simulink model "sampleModel53"  (R2021b)
settings: Solver=VariableStepAuto  StartTime=0.0  StopTime=10.0  RelTol=1e-3
undefined symbols (not defined in the file or in its folder): DiscIntNeverNeededParam, magnitude, Newton, Raphson
libraries: simulink x11, slpidlib x1
settings Model: Creator=user  LastModifiedBy=user

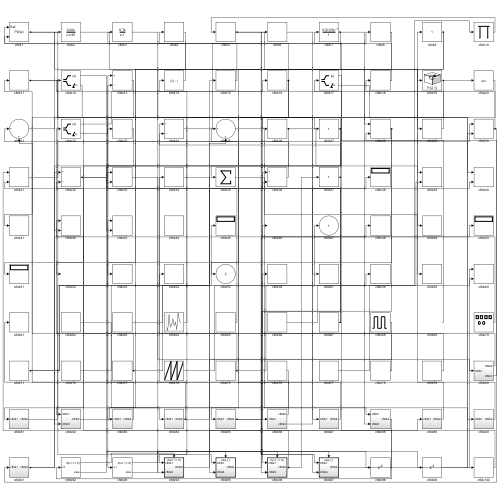
[thumbnail: Simulink's stored preview of the top-level diagram]
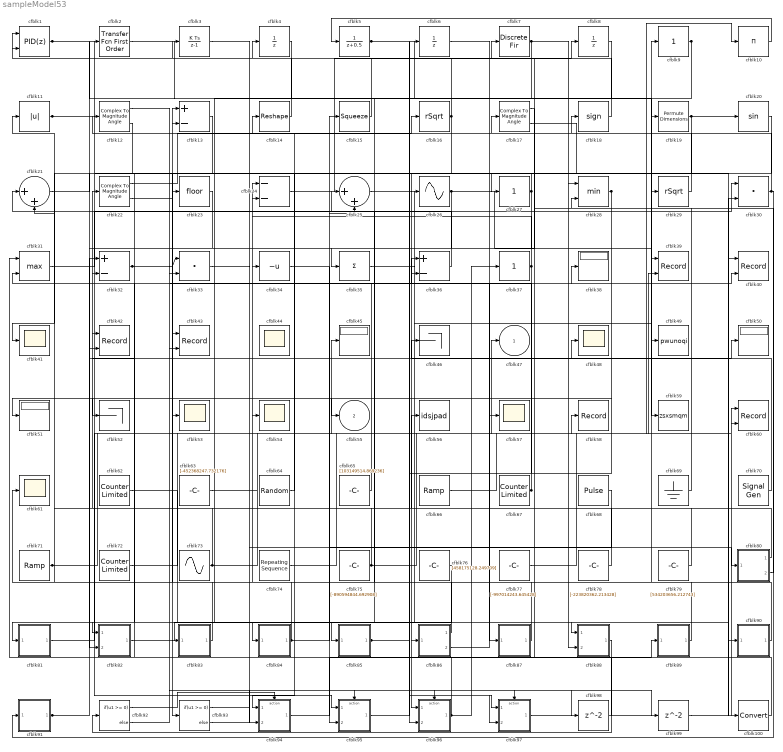
== system sampleModel53 ==
  cfblk1 : slpidlib/PID Controller (2DOF)  Controller=PID  Form=Parallel  TimeDomain=Discrete-time  UseExternalTs=off  SampleTime=1  IntegratorMethod=Forward Euler  FilterMethod=Forward Euler  ControllerParametersSource=internal  P=1  I=1  D=0  UseFilter=on  N=100  b=1  c=1  TunerSelectOption=Transfer Function Based (PID Tuner App)  InitialConditionSource=internal  InitialConditionForIntegrator=0  InitialConditionForFilter=0  DifferentiatorICPrevScaledInput=0  ExternalReset=none  TrackingMode=off  Kt=1  LimitOutput=off  SatLimitsSource=internal  UpperSaturationLimit=inf  LowerSaturationLimit=-inf  LinearizeAsGain=off  AntiWindupMode=none  Kb=1  POutMin=[]  POutMax=[]  IOutMin=[]  IOutMax=[]  DOutMin=[]  DOutMax=[]  NOutMin=[]  NOutMax=[]  bOutMin=[]  bOutMax=[]  cOutMin=[]  cOutMax=[]  SumOutMin=[]  SumOutMax=[]  SaturationOutMin=[]  SaturationOutMax=[]  PParamMin=[]  PParamMax=[]  IParamMin=[]  IParamMax=[]  DParamMin=[]  DParamMax=[]  NParamMin=[]  NParamMax=[]  bParamMin=[]  bParamMax=[]  cParamMin=[]  cParamMax=[]  KbParamMin=[]  KbParamMax=[]  KtParamMin=[]  KtParamMax=[]  KbOutMin=[]  KbOutMax=[]  KtOutMin=[]  KtOutMax=[]  IntegratorOutMin=[]  IntegratorOutMax=[]  FilterOutMin=[]  FilterOutMax=[]  SumI1OutMin=[]  SumI1OutMax=[]  SumI2OutMin=[]  SumI2OutMax=[]  SumI3OutMin=[]  SumI3OutMax=[]  SumI4OutMin=[]  SumI4OutMax=[]  SumDOutMin=[]  SumDOutMax=[]  Sum1OutMin=[]  Sum1OutMax=[]  Sum2OutMin=[]  Sum2OutMax=[]  Sum3OutMin=[]  Sum3OutMax=[]  DifferentiatorOutMin=[]  DifferentiatorOutMax=[]  FilterDiffOutCoefMin=[]  FilterDiffOutCoefMax=[]  ReciprocalOutMin=[]  ReciprocalOutMax=[]  SumDenOutMin=[]  SumDenOutMax=[]  SumNumOutMin=[]  SumNumOutMax=[]  DivideOutMin=[]  DivideOutMax=[]  UdiffTsProdOutMin=[]  UdiffTsProdOutMax=[]  NTsProdOutMin=[]  NTsProdOutMax=[]  UintegralTsProdOutMin=[]  UintegralTsProdOutMax=[]  UngainTsProdOutMin=[]  UngainTsProdOutMax=[]  IntegratorContinuousStateAttributes=''  IntegratorStateMustResolveToSignalObject=off  IntegratorRTWStateStorageClass=Auto  FilterContinuousStateAttributes=''  FilterStateMustResolveToSignalObject=off  FilterRTWStateStorageClass=Auto  ParallelPVariant=InternalParameters  IdealPVariant=Disabled  IVariant=InternalParameters  DVariant=InternalParameters  bVariant=InternalParameters  cVariant=InternalParameters  IntegratorVariant=Discrete  SatVariant=Disabled  AWVariant=Passthrough  PCopyVariant=Disabled  TRVariant=Disabled  FdbkBlocksVariant=Forward  IdealPFdbkVariant=Disabled  SatFdbkVariant=Disabled  DerivativeFilterVariant=ForwardEulerFilter  NVariant=InternalParameters  NCopyVariant=Disabled  FilterICVariant=InternalICsFilter  IntegratorICVariant=InternalICs  ExternalResetVariant=Disabled  TRSumVariant=Passthrough  SumFdbkVariant=Disabled  SumVariant=Sum_PID  TsampFilterVariant=InternalTs  TsampNgainVariant=Passthrough  TsampIntegralVariant=Passthrough  ExternalSaturationOutDataTypeStr=Inherit: Same as second input
      settings: SourceProductBaseCode=SL
  cfblk10 : Product  Inputs=*
  cfblk100 : DataTypeConversion
  cfblk11 : Abs
  cfblk12 : ComplexToMagnitudeAngle
  cfblk13 : Sum  Inputs=+-
  cfblk14 : Reshape
  cfblk15 : Squeeze
  cfblk16 : Sqrt  Operator=rSqrt  AlgorithmType=Newton-Raphson  SaturateOnIntegerOverflow=on
  cfblk17 : ComplexToMagnitudeAngle
  cfblk18 : Signum
  cfblk19 : PermuteDimensions
  cfblk2 : simulink/Discrete/Transfer Fcn First Order  PoleZ=0.95  ICPrevOutput=0.0  DoSatur=off
  cfblk20 : Trigonometry
  cfblk21 : Sum  Inputs=|++
  cfblk22 : ComplexToMagnitudeAngle
  cfblk23 : Rounding
  cfblk24 : Sum  Inputs=--
  cfblk25 : Sum  Inputs=|++
  cfblk26 : Sin  TimeSource=Use external signal  SampleTime=0
  cfblk27 : simulink/Math Operations/Slider Gain  gain=1  low=0  high=2
  cfblk28 : MinMax  Inputs=2
  cfblk29 : Sqrt  Operator=rSqrt  AlgorithmType=Newton-Raphson  SaturateOnIntegerOverflow=on
  cfblk3 : DiscreteIntegrator  ICPrevOutput=DiscIntNeverNeededParam  ICPrevScaledInput=DiscIntNeverNeededParam
  cfblk30 : DotProduct  InputSameDT=on  OutDataTypeStr=Inherit: Inherit via internal rule
  cfblk31 : MinMax  Function=max  Inputs=2
  cfblk32 : Sum  Inputs=+-
  cfblk33 : DotProduct  InputSameDT=on  OutDataTypeStr=Inherit: Inherit via internal rule
  cfblk34 : UnaryMinus
  cfblk35 : Sum  Inputs=+
  cfblk36 : Sum  Inputs=+-
  cfblk37 : simulink/Math Operations/Slider Gain  gain=1  low=0  high=2
  cfblk{38,45,50..51} (4 alike) : Display
  cfblk39 : Record  FileSettingsInternal="{\"entries\":[{\"content\":{\"excelSettings\":{\"content\":{},\"type\":\"Streamout.ExcelSettings\"}},\"type\":\"Streamout.FileSettingStorage\",\"uuid\":\"36555a3f-5799-4d89-b4f4-813525baae06\"}],\"packageUris\":[\"http://schema.mathworks.com/mf0/streamout_blocks/R2020a\"],\"version\":\"1.0\"}"  Layout=[1 1]  SignalsInternal="{\"entries\":[{\"content\":{\"signals\":[{\"content\":{\"blockPath\":[\"sampleModel53/cfblk39\"],\"channel\":[],\"dimensions\":[1],\"domain\":\"sampleModel53/cfblk39\",\"lineColor\":\"#a2142f\",\"plots\":[1],\"port\":1,\"sid\":[\"\"],\"signalID\":2017,\"signalName\":\"cfblk26\"},\"type\":\"RecordBlkView.Signal\",\"uuid\":\"47f0a369-7cc4-4aaa-9385-732514935d38\"},{\"content\":{\"blockPath\":[\"sampleModel53/cfblk39\"],\"channel\":[],\"dimensions\":[1],\"domain\":\"sampleModel53/cfblk39\",\"lineColor\":\"#139fff\",\"plots\":[1],\"port\":2,\"sid\":[\"\"],\"signalID\":2021,\"signalName\":\"cfblk75\"},\"type\":\"RecordBlkView.Signal\",\"uuid\":\"4d1bc853-d276-4e83-93c2-32a1ede8454b\"}]},\"type\":\"RecordBlkView.InputSignals\",\"uuid\":\"ef9d1d75-79a9-4377-b019-a30109193e72\"}],\"packageUris\":[\"http://schema.mathworks.com/mf0/streamout_blocks/R2020a\"],\"version\":\"1.0\"}"  VisualizationBindings="{\"xyplotplugin\":{\"info\":[{\"series\":[{\"bindingParametersList\":[{\"parameter\":\"X-Axis\",\"signalID\":2017,\"signalName\":\"cfblk26\"},{\"parameter\":\"Y-Axis\",\"signalID\":2021,\"signalName\":\"cfblk75\"}],\"seriesID\":35911}],\"subplotID\":1}]}}"  CompatibilityTag=XY
  cfblk4 : UnitDelay  HasFrameUpgradeWarning=on
  cfblk40 : Record  FileSettingsInternal="{\"entries\":[{\"content\":{\"excelSettings\":{\"content\":{},\"type\":\"Streamout.ExcelSettings\"}},\"type\":\"Streamout.FileSettingStorage\",\"uuid\":\"29f311e9-4cb5-4aae-ab6d-f238a6542dbf\"}],\"packageUris\":[\"http://schema.mathworks.com/mf0/streamout_blocks/R2020a\"],\"version\":\"1.0\"}"  Layout=[1 1]  SignalsInternal="{\"entries\":[{\"content\":{\"signals\":[{\"content\":{\"blockPath\":[\"sampleModel53/cfblk40\"],\"channel\":[],\"dimensions\":[1],\"domain\":\"sampleModel53/cfblk40\",\"lineColor\":\"#a2142f\",\"plots\":[1],\"port\":1,\"sid\":[\"\"],\"signalID\":2025,\"signalName\":\"cfblk11\"},\"type\":\"RecordBlkView.Signal\",\"uuid\":\"6599d64e-fdeb-4881-badc-896bf7f9b191\"},{\"content\":{\"blockPath\":[\"sampleModel53/cfblk40\"],\"channel\":[],\"dimensions\":[1],\"domain\":\"sampleModel53/cfblk40\",\"lineColor\":\"#139fff\",\"plots\":[1],\"port\":2,\"sid\":[\"\"],\"signalID\":2029,\"signalName\":\"cfblk32\"},\"type\":\"RecordBlkView.Signal\",\"uuid\":\"6d17c54a-5a2b-4875-95ea-40abd550d686\"}]},\"type\":\"RecordBlkView.InputSignals\",\"uuid\":\"16042054-2248-4dd5-be65-24b2471db457\"}],\"packageUris\":[\"http://schema.mathworks.com/mf0/streamout_blocks/R2020a\"],\"version\":\"1.0\"}"  VisualizationBindings="{\"xyplotplugin\":{\"info\":[{\"series\":[{\"bindingParametersList\":[{\"parameter\":\"X-Axis\",\"signalID\":2025,\"signalName\":\"cfblk11\"},{\"parameter\":\"Y-Axis\",\"signalID\":2029,\"signalName\":\"cfblk32\"}],\"seriesID\":247}],\"subplotID\":1}]}}"  CompatibilityTag=XY
  cfblk{41,44,48,53..54,57,61} (7 alike) : Scope
      cfblk44 settings: Floating=on
  cfblk42 : Record  FileSettingsInternal="{\"entries\":[{\"content\":{\"excelSettings\":{\"content\":{},\"type\":\"Streamout.ExcelSettings\"}},\"type\":\"Streamout.FileSettingStorage\",\"uuid\":\"2795f945-7d6f-4af1-afb2-df17c85014fd\"}],\"packageUris\":[\"http://schema.mathworks.com/mf0/streamout_blocks/R2020a\"],\"version\":\"1.0\"}"  Layout=[1 1]  SignalsInternal="{\"entries\":[{\"content\":{\"signals\":[{\"content\":{\"blockPath\":[\"sampleModel53/cfblk42\"],\"channel\":[],\"dimensions\":[1],\"domain\":\"sampleModel53/cfblk42\",\"lineColor\":\"#a2142f\",\"plots\":[1],\"port\":1,\"sid\":[\"\"],\"signalID\":2033,\"signalName\":\"cfblk96\"},\"type\":\"RecordBlkView.Signal\",\"uuid\":\"f70ba7eb-dc46-4726-8912-a281d005d84a\"},{\"content\":{\"blockPath\":[\"sampleModel53/cfblk42\"],\"channel\":[],\"dimensions\":[1],\"domain\":\"sampleModel53/cfblk42\",\"lineColor\":\"#139fff\",\"plots\":[1],\"port\":2,\"sid\":[\"\"],\"signalID\":2037,\"signalName\":\"cfblk27\"},\"type\":\"RecordBlkView.Signal\",\"uuid\":\"e8cdc3a5-91fa-4319-be48-d51676adf6e4\"}]},\"type\":\"RecordBlkView.InputSignals\",\"uuid\":\"f027bfeb-bbc1-4bf5-989f-a466d2fc895d\"}],\"packageUris\":[\"http://schema.mathworks.com/mf0/streamout_blocks/R2020a\"],\"version\":\"1.0\"}"  VisualizationBindings="{\"xyplotplugin\":{\"info\":[{\"series\":[{\"bindingParametersList\":[{\"parameter\":\"X-Axis\",\"signalID\":2033,\"signalName\":\"cfblk96\"},{\"parameter\":\"Y-Axis\",\"signalID\":2037,\"signalName\":\"cfblk27\"}],\"seriesID\":22493}],\"subplotID\":1}]}}"  CompatibilityTag=XY
  cfblk43 : Record  FileSettingsInternal="{\"entries\":[{\"content\":{\"excelSettings\":{\"content\":{},\"type\":\"Streamout.ExcelSettings\"}},\"type\":\"Streamout.FileSettingStorage\",\"uuid\":\"262fdbcb-1a99-4405-9c28-3705634d857c\"}],\"packageUris\":[\"http://schema.mathworks.com/mf0/streamout_blocks/R2020a\"],\"version\":\"1.0\"}"  Layout=[1 1]  SignalsInternal="{\"entries\":[{\"content\":{\"signals\":[{\"content\":{\"blockPath\":[\"sampleModel53/cfblk43\"],\"channel\":[],\"dimensions\":[1],\"domain\":\"sampleModel53/cfblk43\",\"lineColor\":\"#a2142f\",\"plots\":[1],\"port\":1,\"sid\":[\"\"],\"signalID\":2041,\"signalName\":\"cfblk71\"},\"type\":\"RecordBlkView.Signal\",\"uuid\":\"31af7c79-9017-45d5-9c95-6f76501c4ed0\"},{\"content\":{\"blockPath\":[\"sampleModel53/cfblk43\"],\"channel\":[],\"dimensions\":[1],\"domain\":\"sampleModel53/cfblk43\",\"lineColor\":\"#139fff\",\"plots\":[1],\"port\":2,\"sid\":[\"\"],\"signalID\":2045,\"signalName\":\"cfblk26\"},\"type\":\"RecordBlkView.Signal\",\"uuid\":\"6227f1e4-0aa9-438c-91b2-f1da6c01766f\"}]},\"type\":\"RecordBlkView.InputSignals\",\"uuid\":\"4e3f22c6-0fd5-443b-ac92-023e98c5f6af\"}],\"packageUris\":[\"http://schema.mathworks.com/mf0/streamout_blocks/R2020a\"],\"version\":\"1.0\"}"  VisualizationBindings="{\"xyplotplugin\":{\"info\":[{\"series\":[{\"bindingParametersList\":[{\"parameter\":\"X-Axis\",\"signalID\":2041,\"signalName\":\"cfblk71\"},{\"parameter\":\"Y-Axis\",\"signalID\":2045,\"signalName\":\"cfblk26\"}],\"seriesID\":22878}],\"subplotID\":1}]}}"  CompatibilityTag=XY
  cfblk46 : Terminator
  cfblk49 : ToWorkspace  VariableName=pwunoqi  SaveFormat=Timeseries  SampleTime=-1
  cfblk5 : DiscreteTransferFcn  SampleTime=1
  cfblk52 : Terminator
  cfblk56 : ToWorkspace  VariableName=idsjpad  SaveFormat=Timeseries  SampleTime=-1
  cfblk58 : Record  FileSettingsInternal="{\"entries\":[{\"content\":{\"excelSettings\":{\"content\":{},\"type\":\"Streamout.ExcelSettings\"}},\"type\":\"Streamout.FileSettingStorage\",\"uuid\":\"e85a456c-a740-4745-ba77-d61e779d1d41\"}],\"packageUris\":[\"http://schema.mathworks.com/mf0/streamout_blocks/R2020a\"],\"version\":\"1.0\"}"  SignalsInternal="{\"entries\":[{\"content\":{\"signals\":[{\"content\":{\"blockPath\":[\"sampleModel53/cfblk58\"],\"channel\":[],\"dimensions\":[1,1],\"domain\":\"sampleModel53/cfblk58\",\"lineColor\":\"#0072bd\",\"plots\":[1],\"port\":1,\"sid\":[\"\"],\"signalID\":2049,\"signalName\":\"cfblk85\"},\"type\":\"RecordBlkView.Signal\",\"uuid\":\"17db5c15-ca79-42f1-988a-ac83bc16403a\"}]},\"type\":\"RecordBlkView.InputSignals\",\"uuid\":\"5543be3e-2cf2-4ad7-9ef1-191d5603f8b7\"}],\"packageUris\":[\"http://schema.mathworks.com/mf0/streamout_blocks/R2020a\"],\"version\":\"1.0\"}"  VisualizationBindings="{\"sparklinesplugin\":{\"info\":[{\"bindingParametersList\":[],\"subplotID\":1}]}}"
  cfblk59 : ToWorkspace  VariableName=zsxsmqm  SaveFormat=Timeseries  SampleTime=-1
  cfblk6 : UnitDelay  HasFrameUpgradeWarning=on
  cfblk60 : Record  FileSettingsInternal="{\"entries\":[{\"content\":{\"excelSettings\":{\"content\":{},\"type\":\"Streamout.ExcelSettings\"}},\"type\":\"Streamout.FileSettingStorage\",\"uuid\":\"266a0de7-ebb2-40d2-bb8b-a752c9a132df\"}],\"packageUris\":[\"http://schema.mathworks.com/mf0/streamout_blocks/R2020a\"],\"version\":\"1.0\"}"  Layout=[1 1]  SignalsInternal="{\"entries\":[{\"content\":{\"signals\":[{\"content\":{\"blockPath\":[\"sampleModel53/cfblk60\"],\"channel\":[],\"dimensions\":[1,1],\"domain\":\"sampleModel53/cfblk60\",\"lineColor\":\"#a2142f\",\"plots\":[1],\"port\":1,\"sid\":[\"\"],\"signalID\":2053,\"signalName\":\"cfblk97\"},\"type\":\"RecordBlkView.Signal\",\"uuid\":\"49a729a9-27c5-4996-8fdc-6a282c899358\"},{\"content\":{\"blockPath\":[\"sampleModel53/cfblk60\"],\"channel\":[],\"dimensions\":[1],\"domain\":\"sampleModel53/cfblk60\",\"lineColor\":\"#139fff\",\"plots\":[1],\"port\":2,\"sid\":[\"\"],\"signalID\":2057,\"signalName\":\"cfblk66\"},\"type\":\"RecordBlkView.Signal\",\"uuid\":\"6ac5d0f1-1282-4ff0-ab72-565fc0b345a4\"}]},\"type\":\"RecordBlkView.InputSignals\",\"uuid\":\"cdacac38-5788-4d0c-a38f-7dc9b2a02f40\"}],\"packageUris\":[\"http://schema.mathworks.com/mf0/streamout_blocks/R2020a\"],\"version\":\"1.0\"}"  VisualizationBindings="{\"xyplotplugin\":{\"info\":[{\"series\":[{\"bindingParametersList\":[{\"parameter\":\"X-Axis\",\"signalID\":2053,\"signalName\":\"cfblk97\"},{\"parameter\":\"Y-Axis\",\"signalID\":2057,\"signalName\":\"cfblk66\"}],\"seriesID\":18023}],\"subplotID\":1}]}}"  CompatibilityTag=XY
  cfblk62 : simulink/Sources/Counter Limited  uplimit=[412.000000]  tsamp=-1
  cfblk63 : Constant  Value=[-452368247.732176]  SampleTime=1
  cfblk64 : UniformRandomNumber  Minimum=[-947621677.396505]  Maximum=[4577245631.312114]  Seed=[41948386.000000]  SampleTime=0.1
  cfblk65 : Constant  Value=[103149514.869236]  SampleTime=1
  cfblk66 : simulink/Sources/Ramp  slope=[-8825.450027]  start=[23.823209]  InitialOutput=[549085.262431]
  cfblk67 : simulink/Sources/Counter Limited  uplimit=[704.000000]  tsamp=-1
  cfblk68 : DiscretePulseGenerator  PulseType=Time based  Amplitude=[352690679.292892]  Period=[77561653.661700]  PulseWidth=5  PhaseDelay=[5.000000]
  cfblk69 : Ground
  cfblk7 : DiscreteFir  SampleTime=1
  cfblk70 : SignalGenerator  WaveForm=sawtooth  Amplitude=[-548495900.306508]
  cfblk71 : simulink/Sources/Ramp  slope=[4666.478299]  start=[41.983300]  InitialOutput=[189060.018572]
  cfblk72 : simulink/Sources/Counter Limited  uplimit=[395.000000]  tsamp=-1
  cfblk73 : Sin  Amplitude=[236450243.117325]  Bias=[354333946.592346]  SampleTime=0
  cfblk74 : simulink/Sources/Repeating Sequence  rep_seq_t=[0 2]  rep_seq_y=[-965358426.288802, 477876210.954182]
  cfblk75 : Constant  Value=[-890594844.692908]  SampleTime=1
  cfblk76 : Constant  Value=[458175128.249709]  SampleTime=1
  cfblk77 : Constant  Value=[-997014243.645428]  SampleTime=1
  cfblk78 : Constant  Value=[-223820362.213428]  SampleTime=1
  cfblk79 : Constant  Value=[534203656.212743]  SampleTime=1
  cfblk8 : UnitDelay  HasFrameUpgradeWarning=on
  cfblk80 : Subsystem
  cfblk81 : Subsystem
  cfblk82 : Subsystem
  cfblk83 : Subsystem
  cfblk84 : Subsystem
  cfblk85 : Subsystem
  cfblk86 : Subsystem
  cfblk87 : Subsystem
  cfblk88 : Subsystem
  cfblk89 : Subsystem
  cfblk9 : simulink/Math Operations/Slider Gain  gain=1  low=0  high=2
  cfblk90 : Subsystem
  cfblk91 : Subsystem
  cfblk92 : If  IfExpression=u1 >= 0  SampleTime=1
  cfblk93 : If  IfExpression=u1 >= 0  SampleTime=1
  cfblk94 : Subsystem  TreatAsAtomicUnit=on
  cfblk95 : Subsystem  TreatAsAtomicUnit=on
  cfblk96 : Subsystem  TreatAsAtomicUnit=on
  cfblk97 : Subsystem  TreatAsAtomicUnit=on
  cfblk98 : Delay  SampleTime=1
  cfblk99 : Delay  SampleTime=1
  cfblk47 : Outport
  cfblk55 : Outport  Port=2
  wires:
  cfblk11/1 -> cfblk95/1(cfblk1), cfblk40/1
  cfblk89/1(cfblk2) -> cfblk9/1
  cfblk77/1 -> cfblk10/1
  cfblk9/1 -> cfblk59/1, cfblk53/1
  cfblk16/1 -> cfblk96/1(cfblk1), cfblk52/1, cfblk1/2, cfblk94/1(cfblk1)
  cfblk36/1 -> cfblk21/1
  cfblk75/1 -> cfblk24/1, cfblk39/2
  cfblk74/1 -> cfblk47/1
  cfblk24/1 -> cfblk8/1
  cfblk88/1(cfblk2) -> cfblk92/1
  cfblk35/1 -> cfblk49/1
  cfblk82/1(cfblk2) -> cfblk84/1(cfblk1)
  cfblk67/1 -> cfblk13/1, cfblk36/1
  cfblk76/1 -> cfblk81/1(cfblk1)
  cfblk14/1 -> cfblk1/1
  cfblk31/1 -> cfblk30/1
  cfblk94/1(cfblk2) -> cfblk89/1(cfblk1)
  cfblk73/1 -> cfblk45/1, cfblk32/2
  cfblk25/1 -> cfblk88/1(cfblk1)
  cfblk13/1 -> cfblk93/1
  cfblk28/1 -> cfblk96/2(cfblk5), cfblk51/1
  cfblk79/1 -> cfblk22/1
  cfblk26/1 -> cfblk39/1, cfblk43/2
  cfblk4/1 -> cfblk83/1(cfblk1)
  cfblk7/1 -> cfblk28/1, cfblk94/2(cfblk4)
  cfblk2/1 -> cfblk88/2(cfblk3)
  cfblk29/1 -> cfblk18/1
  cfblk37/1 -> cfblk86/1(cfblk1), cfblk24/2
  cfblk22/1 -> cfblk16/1
  cfblk1/1 -> cfblk87/1(cfblk1), cfblk19/1
  cfblk83/1(cfblk2) -> cfblk13/2
  cfblk64/1 -> cfblk14/1
  cfblk90/1(cfblk2) -> cfblk25/1
  cfblk97/1(cfblk2) -> cfblk60/1
  cfblk27/1 -> cfblk55/1, cfblk42/2, cfblk26/1
  cfblk30/1 -> cfblk91/1(cfblk1), cfblk12/1
  cfblk15/1 -> cfblk3/1
  cfblk5/1 -> cfblk29/1, cfblk97/2(cfblk4)
  cfblk87/1(cfblk2) -> cfblk61/1
  cfblk18/1 -> cfblk4/1
  cfblk69/1 -> cfblk7/1
  cfblk8/1 -> cfblk35/1
  cfblk80/1(cfblk2) -> cfblk56/1
  cfblk71/1 -> cfblk15/1, cfblk43/1
  cfblk85/1(cfblk2) -> cfblk58/1, cfblk97/1(cfblk1)
  cfblk84/1(cfblk2) -> cfblk31/2, cfblk36/2
  cfblk10/1 -> cfblk5/1
  cfblk66/1 -> cfblk60/2
  cfblk19/1 -> cfblk85/1(cfblk1), cfblk20/1
  cfblk6/1 -> cfblk57/1
  cfblk12/2 -> cfblk41/1
  cfblk22/2 -> cfblk23/1
  cfblk72/1 -> cfblk25/2
  cfblk95/1(cfblk2) -> cfblk50/1
  cfblk70/1 -> cfblk46/1
  cfblk32/1 -> cfblk33/1, cfblk40/2
  cfblk86/1(cfblk2) -> cfblk34/1
  cfblk91/1(cfblk2) -> cfblk32/1, cfblk48/1
  cfblk81/1(cfblk2) -> cfblk54/1
  cfblk23/1 -> cfblk82/1(cfblk1)
  cfblk21/1 -> cfblk2/1
  cfblk78/1 -> cfblk11/1
  cfblk68/1 -> cfblk95/2(cfblk4)
  cfblk17/1 -> cfblk33/2
  cfblk80/2(cfblk3) -> cfblk28/2
  cfblk86/2(cfblk4) -> cfblk38/1
  cfblk3/1 -> cfblk27/1
  cfblk33/1 -> cfblk80/1(cfblk1)
  cfblk65/1 -> cfblk21/2
  cfblk96/1(cfblk2) -> cfblk42/1, cfblk37/1
  cfblk63/1 -> cfblk6/1
  cfblk17/2 -> cfblk90/1(cfblk1)
  cfblk20/1 -> cfblk82/2(cfblk5)
  cfblk92/1 -> cfblk94/Action
  cfblk92/2 -> cfblk95/Action
  cfblk93/1 -> cfblk96/Action
  cfblk93/2 -> cfblk97/Action
  cfblk34/1 -> cfblk98/1
  cfblk98/1 -> cfblk31/1
  cfblk12/1 -> cfblk99/1
  cfblk99/1 -> cfblk30/2
  cfblk62/1 -> cfblk100/1
  cfblk100/1 -> cfblk17/1

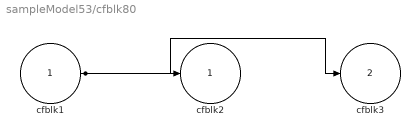
== system sampleModel53/cfblk80 ==
  cfblk1 : Inport
  cfblk2 : Outport
  cfblk3 : Outport  Port=2
  wires:
  cfblk1/1 -> cfblk3/1, cfblk2/1

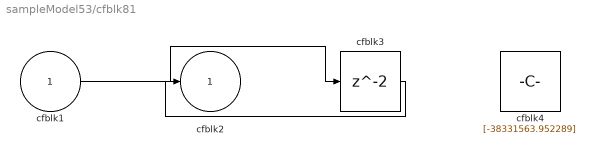
== system sampleModel53/cfblk81 ==
  cfblk1 : Inport
  cfblk3 : Delay  SampleTime=1
  cfblk4 : Constant  Value=[-38331563.952289]  SampleTime=1
  cfblk2 : Outport
  wires:
  cfblk1/1 -> cfblk3/1
  cfblk3/1 -> cfblk2/1

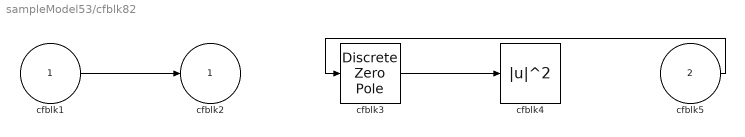
== system sampleModel53/cfblk82 ==
  cfblk1 : Inport
  cfblk5 : Inport  Port=2
  cfblk3 : DiscreteZeroPole  Poles=[0 0.5]  Gain=1
  cfblk4 : Math  Operator=magnitude^2  SaturateOnIntegerOverflow=on
  cfblk2 : Outport
  wires:
  cfblk5/1 -> cfblk3/1
  cfblk1/1 -> cfblk2/1
  cfblk3/1 -> cfblk4/1

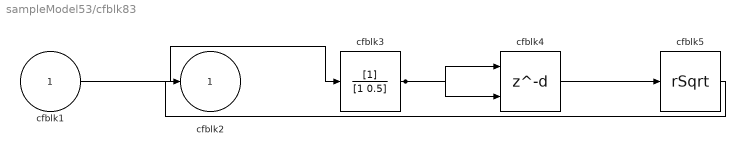
== system sampleModel53/cfblk83 ==
  cfblk1 : Inport
  cfblk3 : DiscreteFilter  SampleTime=1
  cfblk4 : Delay  DelayLengthSource=Input port  SampleTime=1
      settings: InputPortMap=u0,p1
  cfblk5 : Sqrt  Operator=rSqrt  AlgorithmType=Newton-Raphson  SaturateOnIntegerOverflow=on
  cfblk2 : Outport
  wires:
  cfblk1/1 -> cfblk3/1
  cfblk4/1 -> cfblk5/1
  cfblk3/1 -> cfblk4/1, cfblk4/2
  cfblk5/1 -> cfblk2/1

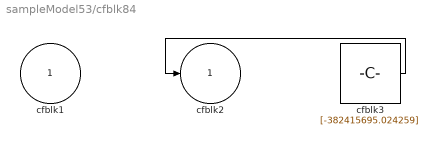
== system sampleModel53/cfblk84 ==
  cfblk1 : Inport
  cfblk3 : Constant  Value=[-382415695.024259]  SampleTime=1
  cfblk2 : Outport
  wires:
  cfblk3/1 -> cfblk2/1

== system sampleModel53/cfblk85 ==
  cfblk1 : Inport
  cfblk3 : Rounding
  cfblk2 : Outport
  wires:
  cfblk3/1 -> cfblk2/1
  cfblk1/1 -> cfblk3/1

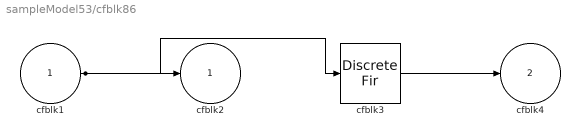
== system sampleModel53/cfblk86 ==
  cfblk1 : Inport
  cfblk3 : DiscreteFir  SampleTime=1
  cfblk2 : Outport
  cfblk4 : Outport  Port=2
  wires:
  cfblk1/1 -> cfblk2/1, cfblk3/1
  cfblk3/1 -> cfblk4/1

== system sampleModel53/cfblk87 ==
  cfblk1 : Inport
  cfblk3 : Constant  Value=[-332438215.445061]  SampleTime=1
  cfblk2 : Outport
  wires:
  cfblk3/1 -> cfblk2/1

== system sampleModel53/cfblk88 ==
  cfblk1 : Inport
  cfblk3 : Inport  Port=2
  cfblk2 : Outport
  wires:
  cfblk3/1 -> cfblk2/1

== system sampleModel53/cfblk89 ==
  cfblk1 : Inport
  cfblk3 : Constant  Value=[-713516553.557210]  SampleTime=1
  cfblk2 : Outport
  wires:
  cfblk1/1 -> cfblk2/1

== system sampleModel53/cfblk90 ==
  cfblk1 : Inport
  cfblk3 : Sum  Inputs=|++
  cfblk2 : Outport
  wires:
  cfblk3/1 -> cfblk2/1
  cfblk1/1 -> cfblk3/1, cfblk3/2

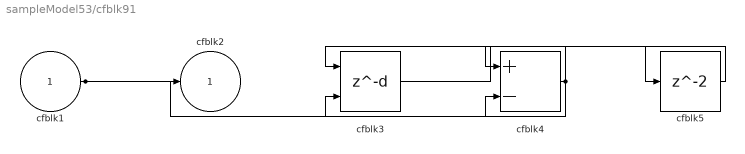
== system sampleModel53/cfblk91 ==
  cfblk1 : Inport
  cfblk3 : Delay  DelayLengthSource=Input port  SampleTime=1
      settings: InputPortMap=u0,p1
  cfblk4 : Sum  Inputs=+-
  cfblk5 : Delay  SampleTime=1
  cfblk2 : Outport
  wires:
  cfblk1/1 -> cfblk4/2, cfblk2/1
  cfblk4/1 -> cfblk3/1, cfblk3/2
  cfblk3/1 -> cfblk5/1
  cfblk5/1 -> cfblk4/1

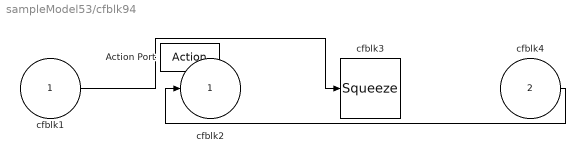
== system sampleModel53/cfblk94 ==
  cfblk1 : Inport
  cfblk4 : Inport  Port=2
  Action Port : ActionPort  ActionPortLabel=if(u1 >= 0)
  cfblk3 : Squeeze
  cfblk2 : Outport
  wires:
  cfblk4/1 -> cfblk2/1
  cfblk1/1 -> cfblk3/1

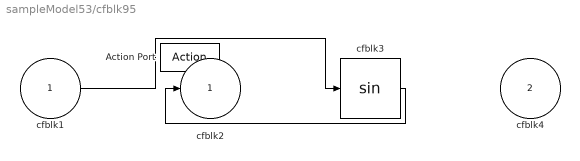
== system sampleModel53/cfblk95 ==
  cfblk1 : Inport
  cfblk4 : Inport  Port=2
  Action Port : ActionPort  ActionPortLabel=else
  cfblk3 : Trigonometry
  cfblk2 : Outport
  wires:
  cfblk3/1 -> cfblk2/1
  cfblk1/1 -> cfblk3/1

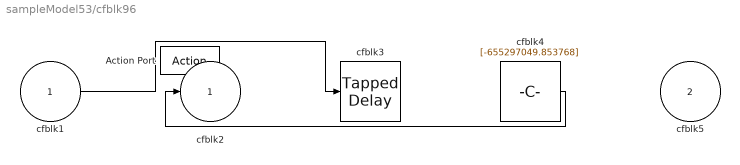
== system sampleModel53/cfblk96 ==
  cfblk1 : Inport
  cfblk5 : Inport  Port=2
  Action Port : ActionPort  ActionPortLabel=if(u1 >= 0)
  cfblk3 : simulink/Discrete/Tapped Delay  vinit=0.0  samptime=-1  NumDelays=1  DelayOrder=Oldest  includeCurrent=off
  cfblk4 : Constant  Value=[-655297049.853768]  SampleTime=1
  cfblk2 : Outport
  wires:
  cfblk4/1 -> cfblk2/1
  cfblk1/1 -> cfblk3/1

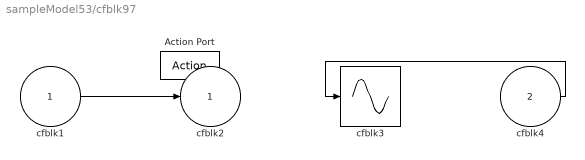
== system sampleModel53/cfblk97 ==
  cfblk1 : Inport
  cfblk4 : Inport  Port=2
  Action Port : ActionPort  ActionPortLabel=else
  cfblk3 : Sin  TimeSource=Use external signal  SampleTime=0
  cfblk2 : Outport
  wires:
  cfblk4/1 -> cfblk3/1
  cfblk1/1 -> cfblk2/1
